simulink model "pil_testing_double_ms_full"  (R2016a)
settings: Solver=FixedStepAuto  StartTime=0.0  StopTime=inf  FixedStep=0.05  RelTol=1e-3
undefined symbols (not defined in the file): Serial_Port, Standard_Devices
libraries: sldrtlib x4
settings Model: SimulationMode=external  Creator=aless  LastModifiedBy=aless
settings SolverCC: EnableConcurrentExecution=on
settings DataIOCC: SaveFormat=StructureWithTime  SignalLogging=off  DSMLogging=off
settings OptimizationCC: BlockReduction=off  DefaultUnderspecifiedDataType=single  OptimizeBlockIOStorage=off  BufferReuse=off  GlobalBufferReuse=off  ExpressionFolding=off  LocalBlockOutputs=off
settings DebuggingCC: MultiTaskRateTransMsg=warning
settings HardwareCC: ProdBitPerLong=64  ProdLargestAtomicFloat=None  ProdHWDeviceType=Intel->x86-64  TargetBitPerLong=64  TargetBitPerPointer=64  TargetIntDivRoundTo=Zero  TargetEndianess=LittleEndian  TargetWordSize=64  TargetHWDeviceType=Intel->x86-64
settings RTWCC: SystemTargetFile=sldrt.tlc  TemplateMakefile=sldrt.tmf  Description=Simulink Desktop Real-Time  RTWVerbose=off  RTWCompilerOptimization=on
settings CodeAppCC: ForceParamTrailComments=on  MaxIdLength=95  OperatorAnnotations=on  MATLABSourceComments=on
settings SimulinkDesktopRealTimeCC: TargetPreCompLibLocation=C:\Program Files\MATLAB\R2016a\toolbox\sldrt\lib\win64  TargetLangStandard=C89/C90 (ANSI)  SupportVariableSizeSignals=off

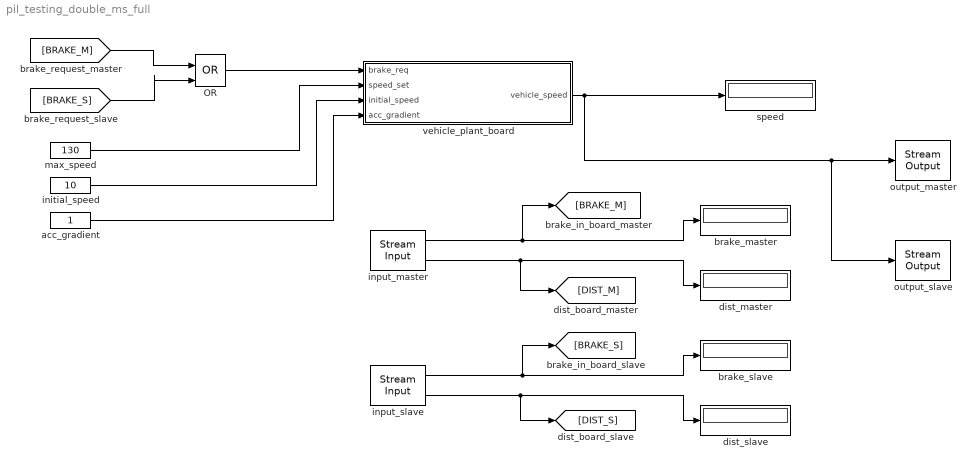
== system pil_testing_double_ms_full ==
  OR : Logic  Operator=OR  IconShape=distinctive  AllPortsSameDT=off  OutDataTypeStr=boolean
  acc_gradient : Constant
  brake_master : Display
  brake_slave : Display
  dist_master : Display
  dist_slave : Display
  initial_speed : Constant  Value=10
  input_master : sldrtlib/Stream Input  SampleTime=0.1  MaxMissedTicks=10  ShowMissedTicks=off  YieldWhenWaiting=off  DrvName=Standard_Devices/Serial_Port  DrvAddress=5  DrvOptions=[9600 8 0 0 0 0 0 0]  DataTypes={'uint8','uint8'}  FormatString='%d %d'  Terminator='\n'  ShowReady=off  ShowError=off
      settings: AttributesFormatString=Standard Devices\nSerial Port [5h]
  input_slave : sldrtlib/Stream Input  SampleTime=0.1  MaxMissedTicks=10  ShowMissedTicks=off  YieldWhenWaiting=off  DrvName=Standard_Devices/Serial_Port  DrvAddress=8  DrvOptions=[9600 8 0 0 0 0 0 0]  DataTypes={'uint8','uint8'}  FormatString='%d %d'  Terminator='\n'  ShowReady=off  ShowError=off
      settings: AttributesFormatString=Standard Devices\nSerial Port [8h]
  max_speed : Constant  Value=130
  output_master : sldrtlib/Stream Output  SampleTime=0.1  MaxMissedTicks=10  ShowMissedTicks=off  YieldWhenWaiting=off  DrvName=Standard_Devices/Serial_Port  DrvAddress=5  DrvOptions=[9600 8 0 0 0 0 0 0]  PortSizes=1  FormatString='%d\r'  ShowReady=off  ShowError=off  InitialValue=[]  FinalValue=[]
      settings: AttributesFormatString=Standard Devices\nSerial Port [5h]
  output_slave : sldrtlib/Stream Output  SampleTime=0.1  MaxMissedTicks=10  ShowMissedTicks=off  YieldWhenWaiting=off  DrvName=Standard_Devices/Serial_Port  DrvAddress=8  DrvOptions=[9600 8 0 0 0 0 0 0]  PortSizes=1  FormatString='%d\r'  ShowReady=off  ShowError=off  InitialValue=[]  FinalValue=[]
      settings: AttributesFormatString=Standard Devices\nSerial Port [8h]
  speed : Display
  vehicle_plant_board : Subsystem
  wires:
  max_speed/1 -> vehicle_plant_board/2(speed_set)
  initial_speed/1 -> vehicle_plant_board/3(initial_speed)
  acc_gradient/1 -> vehicle_plant_board/4(acc_gradient)
  input_master/1 -> [BRAKE_M], brake_master/1
  input_master/2 -> dist_master/1, [DIST_M]
  vehicle_plant_board/1(vehicle_speed) -> output_slave/1, output_master/1, speed/1
  input_slave/1 -> [BRAKE_S], brake_slave/1
  input_slave/2 -> dist_slave/1, [DIST_S]
  OR/1 -> vehicle_plant_board/1(brake_req)
  [BRAKE_M] -> OR/1
  [BRAKE_S] -> OR/2

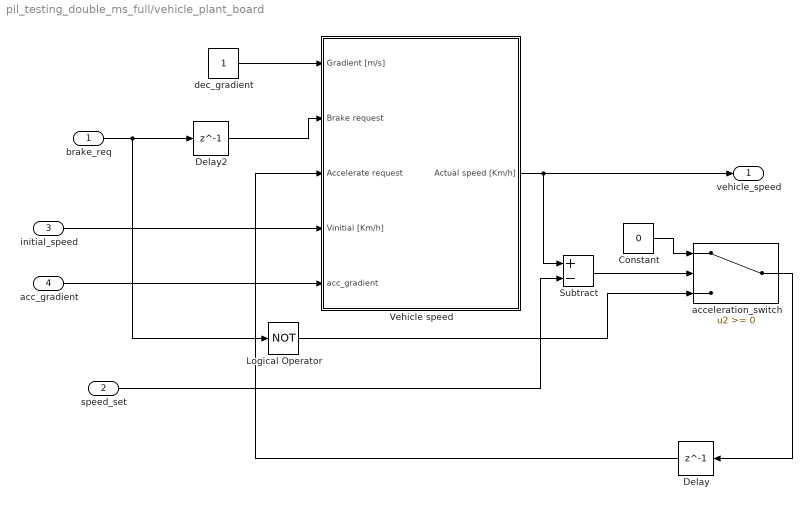
== system pil_testing_double_ms_full/vehicle_plant_board ==
  brake_req : Inport
  speed_set : Inport  Port=2
  initial_speed : Inport  Port=3
  acc_gradient : Inport  Port=4
  Constant : Constant  Value=0
  Delay : Delay  DelayLength=1  InitialCondition=0
  Delay2 : Delay  DelayLength=1  InitialCondition=0
  Logical Operator : Logic  Operator=NOT  AllPortsSameDT=off  OutDataTypeStr=boolean
  Subtract : Sum  Inputs=+-
  Vehicle speed : Subsystem
  acceleration_switch : Switch  RndMeth=Nearest
  dec_gradient : Constant
  vehicle_speed : Outport
  wires:
  dec_gradient/1 -> Vehicle speed/1(Gradient [m/s])
  initial_speed/1 -> Vehicle speed/4(Vinitial [Km/h])
  Vehicle speed/1(Actual speed [Km/h]) -> vehicle_speed/1, Subtract/1
  Constant/1 -> acceleration_switch/1
  brake_req/1 -> Logical Operator/1, Delay2/1
  acceleration_switch/1 -> Delay/1
  Subtract/1 -> acceleration_switch/2
  speed_set/1 -> Subtract/2
  Delay2/1 -> Vehicle speed/2(Brake request)
  Logical Operator/1 -> acceleration_switch/3
  acc_gradient/1 -> Vehicle speed/5(acc_gradient)
  Delay/1 -> Vehicle speed/3(Accelerate request)

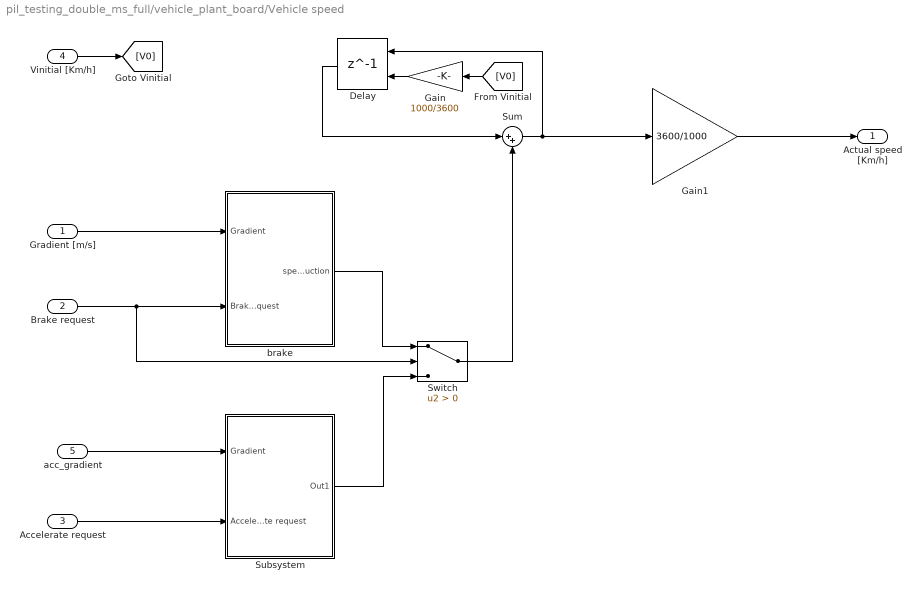
== system pil_testing_double_ms_full/vehicle_plant_board/Vehicle speed ==
  Gradient [m/s] : Inport
  Brake request : Inport  Port=2
  Accelerate request : Inport  Port=3
  Vinitial [Km/h] : Inport  Port=4
  acc_gradient : Inport  Port=5
  Delay : Delay  DelayLength=1  InitialConditionSource=Input port  InitialCondition=0
      settings: InputPortMap=u0,p4
  Gain : Gain  Gain=1000/3600
  Gain1 : Gain  Gain=3600/1000
  Subsystem : Subsystem
  Sum : Sum  Inputs=|++
  Switch : Switch  Criteria=u2 > Threshold
  brake : Subsystem
  Actual speed [Km/h] : Outport
  wires:
  Brake request/1 -> Switch/2, brake/2(Brake request)
  Gradient [m/s]/1 -> brake/1(Gradient)
  Gain/1 -> Delay/2
  Subsystem/1(Out1) -> Switch/3
  Gain1/1 -> Actual speed [Km/h]/1
  Switch/1 -> Sum/2
  Accelerate request/1 -> Subsystem/2(Acceleate request)
  brake/1(speed_reduction) -> Switch/1
  Sum/1 -> Gain1/1, Delay/1
  [V0] -> Gain/1
  Delay/1 -> Sum/1
  Vinitial [Km/h]/1 -> [V0]
  acc_gradient/1 -> Subsystem/1(Gradient)

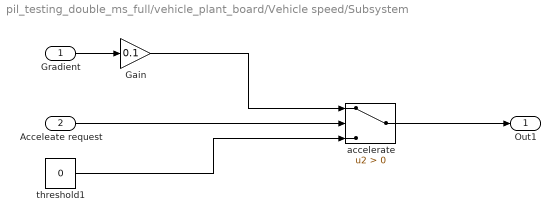
== system pil_testing_double_ms_full/vehicle_plant_board/Vehicle speed/Subsystem ==
  Gradient : Inport
  Acceleate request : Inport  Port=2
  Gain : Gain  Gain=0.1
  accelerate : Switch  Criteria=u2 > Threshold
  threshold1 : Constant  Value=0
  Out1 : Outport
  wires:
  accelerate/1 -> Out1/1
  Acceleate request/1 -> accelerate/2
  Gradient/1 -> Gain/1
  threshold1/1 -> accelerate/3
  Gain/1 -> accelerate/1

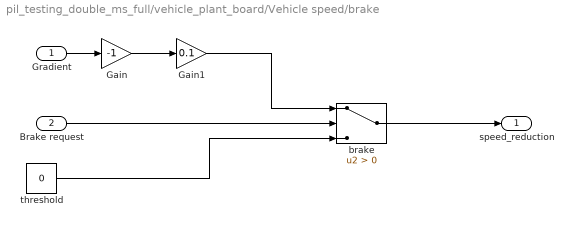
== system pil_testing_double_ms_full/vehicle_plant_board/Vehicle speed/brake ==
  Gradient : Inport
  Brake request : Inport  Port=2
  Gain : Gain  Gain=-1
  Gain1 : Gain  Gain=0.1
  brake : Switch  Criteria=u2 > Threshold
  threshold : Constant  Value=0
  speed_reduction : Outport
  wires:
  Gain/1 -> Gain1/1
  Gradient/1 -> Gain/1
  Gain1/1 -> brake/1
  Brake request/1 -> brake/2
  threshold/1 -> brake/3
  brake/1 -> speed_reduction/1
